simulink model "TestMotorOSEK"  (Simulink 6.4)
settings: Solver=FixedStepDiscrete  SolverMode=SingleTasking  StartTime=0  StopTime=inf  FixedStep=0.001  RelTol=1e-3
libraries: ecrobot_nxt_lib x7
settings Model: Creator=tchikama  LastModifiedBy=tchikama  ProdHWDeviceType=ARM7
settings DataIOCC: SaveOutput=off  SignalLogging=off  SaveTime=off
settings OptimizationCC: InlineParams=on  InlineInvariantSignals=on  RollThreshold=2  StateBitsets=on  DataBitsets=on  UseTempVars=on  InitFltsAndDblsToZero=off  NoFixptDivByZeroProtection=on  EfficientFloat2IntCast=on  OptimizeModelRefInitCode=on  LifeSpan=1
settings DebuggingCC: ConsistencyChecking=warning  SignalInfNanChecking=warning  ReadBeforeWriteMsg=DisableAll  WriteAfterWriteMsg=DisableAll  WriteAfterReadMsg=DisableAll  AlgebraicLoopMsg=error  CheckExecutionContextPreStartOutputMsg=on  CheckExecutionContextRuntimeOutputMsg=on  SolverPrmCheckMsg=none  SingleTaskRateTransMsg=warning  TasksWithSamePriorityMsg=none  IntegerOverflowMsg=error  ParameterPrecisionLossMsg=none  UnconnectedInputMsg=error  UnconnectedOutputMsg=error  UnconnectedLineMsg=error  UniqueDataStoreMsg=error  BusObjectLabelMismatch=error  RootOutportRequireBusObject=error  ModelReferenceIOMsg=warning  ModelReferenceVersionMismatchMessage=warning  ModelReferenceIOMismatchMessage=warning
settings HardwareCC: ProdIntDivRoundTo=Zero  ProdEndianess=LittleEndian  ProdHWDeviceType=ARM7  TargetHWDeviceType=32-bit Generic
settings ModelReferenceCC: ModelReferenceNumInstancesAllowed=Single
settings RTWCC: SystemTargetFile=ert.tlc  GenCodeOnly=on  GenerateMakefile=off  TemplateMakefile=ert_default_tmf  Description=Real-Time Workshop Embedded Coder (no auto configuration)  GenerateReport=on  RTWVerbose=off  ProcessScript=ert_make_rtw_hook  IncludeHyperlinkInReport=on  LaunchReport=on
settings CodeAppCC: ForceParamTrailComments=on  IgnoreCustomStorageClasses=off  SFDataObjDesc=on  PrefixModelToSubsysFcnNames=off  CustomSymbolStrGlobalVar=rt$N$M  CustomSymbolStrType=$N$M  CustomSymbolStrFcn=$N$M$F  CustomSymbolStrMacro=$N$M  InsertBlockDesc=on
settings ERTTargetCC: TargetFcnLib=ansi_tfl_tmw.mat  GenFloatMathFcnCalls=GNU  IncludeMdlTerminateFcn=off  SuppressErrorStatus=on  IncludeERTFirstTime=on  SupportAbsoluteTime=off  SupportNonFinite=off  SupportComplex=off  PurelyIntegerCode=on  InlinedParameterPlacement=NonHierarchical  RootIOFormat=Structure reference  ERTCustomFileTemplate=example_file_process.tlc  InitialValueSource=Model

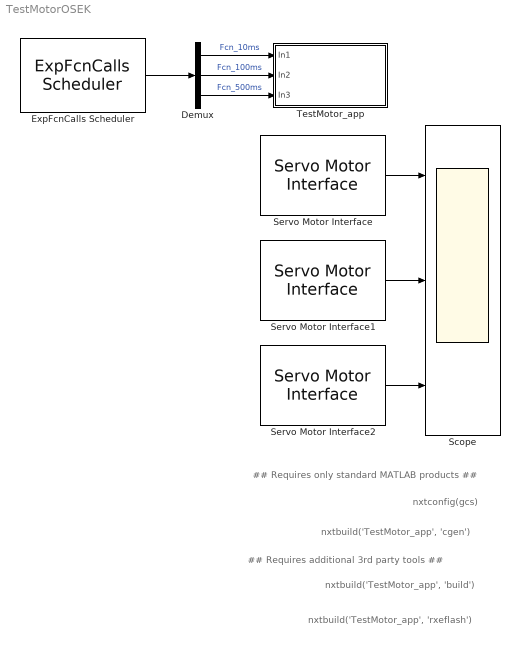
== system TestMotorOSEK ==
  note: nxtbuild('TestMotor_app', 'build')
  note: nxtbuild('TestMotor_app', 'rxeflash')
  note: nxtbuild('TestMotor_app', 'cgen')
  note: ## Requires only standard MATLAB products ##
  note: ## Requires additional 3rd party tools ##
  note: nxtconfig(gcs)
  Demux : Demux  Outputs=3
  ExpFcnCalls Scheduler : ecrobot_nxt_lib/ExpFcnCalls Scheduler  fcname='Fcn_10ms', 'Fcn_100ms', 'Fcn_500ms'  fctrigger=[10 100 500]  ts=0.001  platform=OSEK  stacksize=[64 64 64]  bd_mode=Slave
  Scope : Scope  NumInputPorts=3
      settings: YMin=-100~-100~-100  YMax=100~100~100
  Servo Motor Interface : ecrobot_nxt_lib/Servo Motor Interface  SystemSampleTime=-1  ip=A  mode=Brake
  Servo Motor Interface1 : ecrobot_nxt_lib/Servo Motor Interface  SystemSampleTime=-1  ip=B  mode=Brake
  Servo Motor Interface2 : ecrobot_nxt_lib/Servo Motor Interface  SystemSampleTime=-1  ip=C  mode=Brake
  TestMotor_app : Subsystem
  wires:
  Servo Motor Interface/1 -> Scope/1
  Servo Motor Interface1/1 -> Scope/2
  Servo Motor Interface2/1 -> Scope/3
  ExpFcnCalls Scheduler/1 -> Demux/1
  Demux/1 -> TestMotor_app/1(In1)  "Fcn_10ms"
  Demux/2 -> TestMotor_app/2(In2)  "Fcn_100ms"
  Demux/3 -> TestMotor_app/3(In3)  "Fcn_500ms"

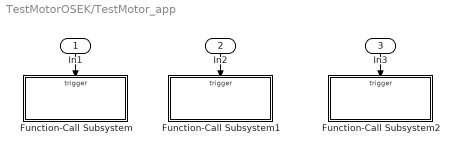
== system TestMotorOSEK/TestMotor_app ==
  In1 : Inport  Orientation=down
  In2 : Inport  Orientation=down  Port=2
  In3 : Inport  Orientation=down  Port=3
  Function-Call Subsystem : Subsystem  TreatAsAtomicUnit=on
  Function-Call Subsystem1 : Subsystem  TreatAsAtomicUnit=on
  Function-Call Subsystem2 : Subsystem  TreatAsAtomicUnit=on
  wires:
  In1/1 -> Function-Call Subsystem/Trigger
  In2/1 -> Function-Call Subsystem1/Trigger
  In3/1 -> Function-Call Subsystem2/Trigger

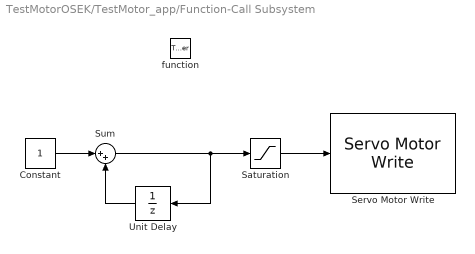
== system TestMotorOSEK/TestMotor_app/Function-Call Subsystem ==
  function : TriggerPort  TriggerType=function-call
  Constant : Constant  Value=1  OutDataTypeMode=int8  OutDataType=sfix(16)  ConRadixGroup=Use specified scaling  OutScaling=2^0  SampleTime=inf  FramePeriod=inf
  Saturation : Saturate  UpperLimit=100  LowerLimit=-100
  Servo Motor Write : ecrobot_nxt_lib/Servo Motor Write  SystemSampleTime=-1  ip=A
  Sum : Sum  Inputs=|++
  Unit Delay : UnitDelay  Orientation=left  SampleTime=-1
  wires:
  Saturation/1 -> Servo Motor Write/1
  Unit Delay/1 -> Sum/2
  Sum/1 -> Saturation/1, Unit Delay/1
  Constant/1 -> Sum/1

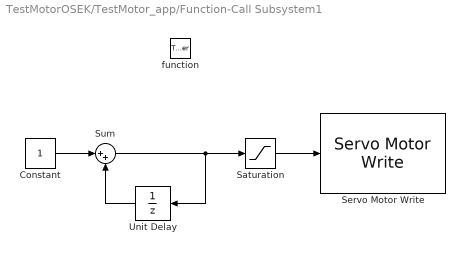
== system TestMotorOSEK/TestMotor_app/Function-Call Subsystem1 ==
  function : TriggerPort  TriggerType=function-call
  Constant : Constant  Value=1  OutDataTypeMode=int8  OutDataType=sfix(16)  ConRadixGroup=Use specified scaling  OutScaling=2^0  SampleTime=inf  FramePeriod=inf
  Saturation : Saturate  UpperLimit=100  LowerLimit=-100
  Servo Motor Write : ecrobot_nxt_lib/Servo Motor Write  SystemSampleTime=-1  ip=B
  Sum : Sum  Inputs=|++
  Unit Delay : UnitDelay  Orientation=left  SampleTime=-1
  wires:
  Constant/1 -> Sum/1
  Sum/1 -> Unit Delay/1, Saturation/1
  Unit Delay/1 -> Sum/2
  Saturation/1 -> Servo Motor Write/1

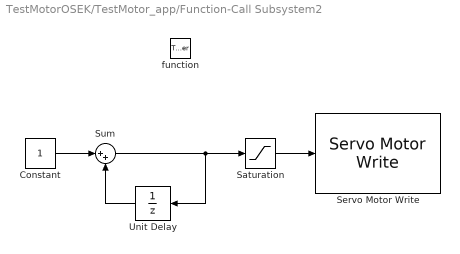
== system TestMotorOSEK/TestMotor_app/Function-Call Subsystem2 ==
  function : TriggerPort  TriggerType=function-call
  Constant : Constant  Value=1  OutDataTypeMode=int8  OutDataType=sfix(16)  ConRadixGroup=Use specified scaling  OutScaling=2^0  SampleTime=inf  FramePeriod=inf
  Saturation : Saturate  UpperLimit=100  LowerLimit=-100
  Servo Motor Write : ecrobot_nxt_lib/Servo Motor Write  SystemSampleTime=-1  ip=C
  Sum : Sum  Inputs=|++
  Unit Delay : UnitDelay  Orientation=left  SampleTime=-1
  wires:
  Saturation/1 -> Servo Motor Write/1
  Unit Delay/1 -> Sum/2
  Sum/1 -> Saturation/1, Unit Delay/1
  Constant/1 -> Sum/1
